simulink model "aero_guidance_airframe"  (Simulink 6.0)
settings: Solver=ode45  SolverMode=SingleTasking  StartTime=0.0  StopTime=10.0  RelTol=1e-3  AbsTol=1e-6
PreLoadFcn:
  | aero_guid_dat
values from neighbouring files (symbols this model uses):
  alpha_vec = [-20:1:20]'*d2r    [aero_guid_dat.m]
  Cm_el = -0.206000/d2r    (= -11.8029305797)    [aero_guid_dat.m]
  Cm_q = -1.719    [aero_guid_dat.m]
  Cz_el = -0.034000/d2r    (= -1.94805650344)    [aero_guid_dat.m]
  d_ref = 0.75/m2ft    (= 0.228599992685)    [aero_guid_dat.m]
  g = 9.81    [aero_guid_dat.m]    (also in aero_raddat.m = 32.2; f14dat.m = 32.2; f14dat_digital.m = 32.2)
  h_ini = 10000/m2ft    (= 3047.99990246)    [aero_guid_dat.m]    (also in aero_lin_aero.m = 10000/m2ft)
  Mach_vec = [2:0.5:4]    [aero_guid_dat.m]
  S_ref = 0.44/m2ft^2    (= 0.0408773349839)    [aero_guid_dat.m]
  Thrust = 10e3    (= 10000)    [aero_guid_dat.m]
  x_ini = 0    [aero_guid_dat.m]
libraries: aerospace x3, simulink x3
settings Model: Creator=The MathWorks Inc.  LastModifiedBy=batserve  ExtModeTrigMode=oneshot  ExtModeArmWhenConnect=off  ExtModeAutoUpdateStatusClock=off
settings DataIOCC: LimitDataPoints=off  SignalLoggingName=logsOut
settings OptimizationCC: BlockReduction=off  BooleanDataType=off
settings DebuggingCC: CheckExecutionContextPreStartOutputMsg=on  CheckExecutionContextRuntimeOutputMsg=on  SolverPrmCheckMsg=none
settings HardwareCC: TargetUnknown=on
settings ModelReferenceCC: UpdateModelReferenceTargets=IfOutOfDate

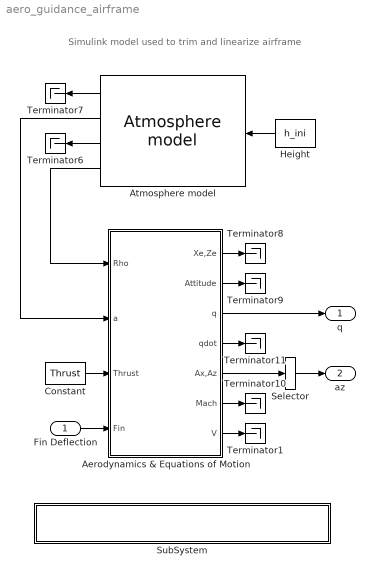
== system aero_guidance_airframe ==
  note: Simulink model used to trim and linearize airframe
  Fin Deflection : Inport  Port=1  LatchInput=off
  Aerodynamics & Equations of Motion : Subsystem  PropExecContextAcrossSSBoundary=on
  Atmosphere model : aerospace/Atmosphere/Atmosphere model  Orientation=left
  Constant : Constant  Value=Thrust
  Height : Constant  Orientation=left  Value=h_ini
  Selector : Selector  Elements=[2]  InputPortWidth=2
  SubSystem : Subsystem  PropExecContextAcrossSSBoundary=on
      settings: OpenFcn=aero_lin_aero
      mask Display: disp('Double-click here to generate linearizations')
  Terminator{1,6..11} (7 alike) : Terminator
  q : Outport  InitialOutput=0
  az : Outport  Port=2  InitialOutput=0
  wires:
  Height/1 -> Atmosphere model/1
  Atmosphere model/1 -> Terminator7/1
  Atmosphere model/3 -> Terminator6/1
  Constant/1 -> Aerodynamics & Equations of Motion/3(Thrust)
  Fin Deflection/1 -> Aerodynamics & Equations of Motion/4(Fin)
  Aerodynamics & Equations of Motion/1(Xe,Ze) -> Terminator8/1
  Aerodynamics & Equations of Motion/2(Attitude) -> Terminator9/1
  Aerodynamics & Equations of Motion/3(q) -> q/1
  Aerodynamics & Equations of Motion/4(qdot) -> Terminator11/1
  Aerodynamics & Equations of Motion/5(Ax,Az) -> Selector/1
  Aerodynamics & Equations of Motion/6(Mach) -> Terminator10/1
  Aerodynamics & Equations of Motion/7(V) -> Terminator1/1
  Atmosphere model/4 -> Aerodynamics & Equations of Motion/1(Rho)
  Atmosphere model/2 -> Aerodynamics & Equations of Motion/2(a)
  Selector/1 -> az/1

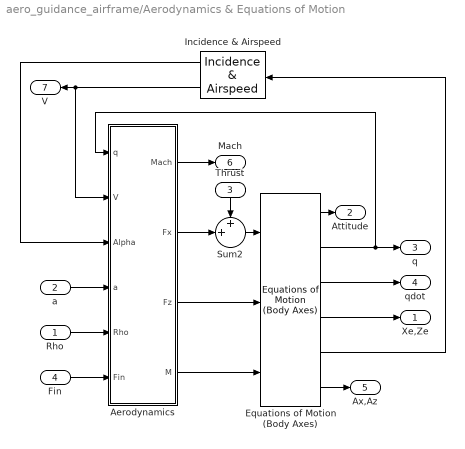
== system aero_guidance_airframe/Aerodynamics & Equations of Motion ==
  Rho : Inport  Port=1  LatchInput=off
  a : Inport  Port=2  LatchInput=off
  Thrust : Inport  Orientation=down  Port=3  LatchInput=off
  Fin : Inport  Port=4  LatchInput=off
  " Equations of Motion (Body Axes)" : aerospace/3DoF Equations of Motion / Equations of Motion (Body Axes)  v_ini=v_ini  theta_ini=theta_ini  alpha_ini=alpha_ini  q_ini=q_ini  pos_ini=[x_ini -h_ini]  mass=mass  Iyy=Iyy  g=g
  Aerodynamics : Subsystem  PropExecContextAcrossSSBoundary=on
  Incidence & Airspeed : aerospace/3DoF Equations of Motion /Incidence  & Airspeed  Orientation=left
  Sum2 : Sum  Inputs=++|  SaturateOnIntegerOverflow=on  InputSameDT=on
  Xe,Ze : Outport  InitialOutput=0
  Attitude : Outport  Port=2  InitialOutput=0
  q : Outport  Port=3  InitialOutput=0
  qdot : Outport  Port=4  InitialOutput=0
  Ax,Az : Outport  Port=5  InitialOutput=0
  Mach : Outport  Port=6  InitialOutput=0
  V : Outport  Orientation=left  Port=7  InitialOutput=0
  wires:
  " Equations of Motion (Body Axes)"/5 -> Incidence & Airspeed/1
  " Equations of Motion (Body Axes)"/6 -> Ax,Az/1
  " Equations of Motion (Body Axes)"/4 -> Xe,Ze/1
  " Equations of Motion (Body Axes)"/1 -> Attitude/1
  " Equations of Motion (Body Axes)"/3 -> qdot/1
  " Equations of Motion (Body Axes)"/2 -> Aerodynamics/1(q), q/1
  Thrust/1 -> Sum2/1
  Aerodynamics/2(Fx) -> Sum2/2
  Aerodynamics/3(Fz) -> " Equations of Motion (Body Axes)"/2
  Incidence & Airspeed/2 -> Aerodynamics/2(V), V/1
  Fin/1 -> Aerodynamics/6(Fin)
  a/1 -> Aerodynamics/4(a)
  Rho/1 -> Aerodynamics/5(Rho)
  Incidence & Airspeed/1 -> Aerodynamics/3(Alpha)
  Sum2/1 -> " Equations of Motion (Body Axes)"/1
  Aerodynamics/4(" M") -> " Equations of Motion (Body Axes)"/3
  Aerodynamics/1(" Mach") -> Mach/1

== system aero_guidance_airframe/SubSystem ==

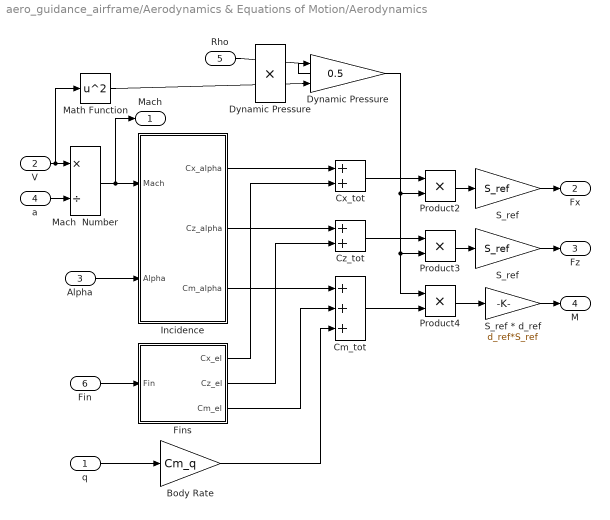
== system aero_guidance_airframe/Aerodynamics & Equations of Motion/Aerodynamics ==
  q : Inport  Port=1  LatchInput=off
  V : Inport  Port=2  LatchInput=off
  Alpha : Inport  Port=3  LatchInput=off
  a : Inport  Port=4  LatchInput=off
  Rho : Inport  Port=5  LatchInput=off
  Fin : Inport  Port=6  LatchInput=off
  Body Rate : Gain  Gain=Cm_q  SaturateOnIntegerOverflow=on
  Cm_tot : Sum  Inputs=+++  SaturateOnIntegerOverflow=on  InputSameDT=on
  Cx_tot : Sum  SaturateOnIntegerOverflow=on  InputSameDT=on
  Cz_tot : Sum  SaturateOnIntegerOverflow=on  InputSameDT=on
  Dynamic Pressure : Gain  Gain=0.5  SaturateOnIntegerOverflow=on
  Dynamic Pressure : Product  SaturateOnIntegerOverflow=on  RndMeth=Zero  InputSameDT=on
  Fins : Subsystem  PropExecContextAcrossSSBoundary=on
  Incidence : Subsystem  PropExecContextAcrossSSBoundary=on
  Mach  Number : Product  Inputs=*/  SaturateOnIntegerOverflow=on  RndMeth=Zero  InputSameDT=on
  Math Function : Math  Operator=square  SaturateOnIntegerOverflow=on
  Product2 : Product  SaturateOnIntegerOverflow=on  RndMeth=Zero  InputSameDT=on
  Product3 : Product  SaturateOnIntegerOverflow=on  RndMeth=Zero  InputSameDT=on
  Product4 : Product  SaturateOnIntegerOverflow=on  RndMeth=Zero  InputSameDT=on
  S_ref : Gain  Gain=S_ref  SaturateOnIntegerOverflow=on
  S_ref * d_ref : Gain  Gain=d_ref*S_ref  SaturateOnIntegerOverflow=on
  "S_ref " : Gain  Gain=S_ref  SaturateOnIntegerOverflow=on
  " Mach" : Outport  InitialOutput=0
  Fx : Outport  Port=2  InitialOutput=[0]
  Fz : Outport  Port=3  InitialOutput=0
  " M" : Outport  Port=4  InitialOutput=0
  wires:
  Mach  Number/1 -> " Mach"/1, Incidence/1(Mach)
  q/1 -> Body Rate/1
  Cm_tot/1 -> Product4/2
  Product4/1 -> S_ref * d_ref/1
  S_ref * d_ref/1 -> " M"/1
  Fin/1 -> Fins/1(Fin)
  "S_ref "/1 -> Fz/1
  Product3/1 -> "S_ref "/1
  S_ref/1 -> Fx/1
  Product2/1 -> S_ref/1
  Cz_tot/1 -> Product3/1
  Cx_tot/1 -> Product2/1
  Alpha/1 -> Incidence/2(Alpha)
  a/1 -> Mach  Number/2
  Body Rate/1 -> Cm_tot/3
  Fins/3(Cm_el) -> Cm_tot/2
  Incidence/3(Cm_alpha) -> Cm_tot/1
  Fins/2(Cz_el) -> Cz_tot/2
  Incidence/2(Cz_alpha) -> Cz_tot/1
  Fins/1(Cx_el) -> Cx_tot/2
  Incidence/1(Cx_alpha) -> Cx_tot/1
  V/1 -> Mach  Number/1, Math Function/1
  Dynamic Pressure/1 -> Product4/1, Product3/2, Product2/2
  Dynamic Pressure/1 -> Dynamic Pressure/1
  Rho/1 -> Dynamic Pressure/1
  Math Function/1 -> Dynamic Pressure/2

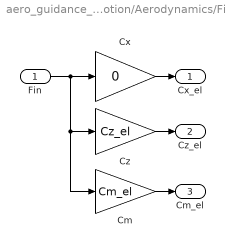
== system aero_guidance_airframe/Aerodynamics & Equations of Motion/Aerodynamics/Fins ==
  Fin : Inport  Port=1  LatchInput=off
  Cm : Gain  Gain=Cm_el  SaturateOnIntegerOverflow=on
  Cx : Gain  Gain=0  SaturateOnIntegerOverflow=on
  Cz : Gain  Gain=Cz_el  SaturateOnIntegerOverflow=on
  Cx_el : Outport  InitialOutput=0
  Cz_el : Outport  Port=2  InitialOutput=0
  Cm_el : Outport  Port=3  InitialOutput=0
  wires:
  Cz/1 -> Cz_el/1
  Cm/1 -> Cm_el/1
  Cx/1 -> Cx_el/1
  Fin/1 -> Cz/1, Cm/1, Cx/1

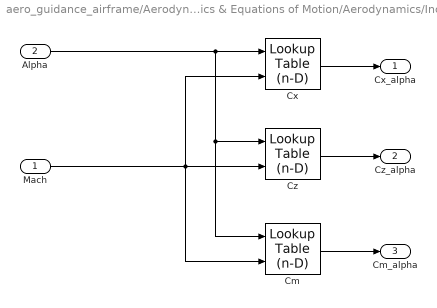
== system aero_guidance_airframe/Aerodynamics & Equations of Motion/Aerodynamics/Incidence ==
  Mach : Inport  Port=1  LatchInput=off
  Alpha : Inport  Port=2  LatchInput=off
  Cm : simulink/Lookup Tables/Lookup Table (n-D)  numDimsPopupSelect=2  bp1=alpha_vec  bp2=Mach_vec  bp3=[1:3]  bp4=[1:3]  bpcell={ [1:3], [1:3] }  explicitNumDims=2  searchMode=Binary Search  cacheBpFlag=on  vectorInputFlag=off  tableData=Cm_alpha  interpMethod=Linear  extrapMethod=Linear  rangeErrorMode=None
  Cx : simulink/Lookup Tables/Lookup Table (n-D)  numDimsPopupSelect=2  bp1=alpha_vec  bp2=Mach_vec  bp3=[1:3]  bp4=[1:3]  bpcell={ [1:3], [1:3] }  explicitNumDims=2  searchMode=Binary Search  cacheBpFlag=on  vectorInputFlag=off  tableData=Cx_alpha  interpMethod=Linear  extrapMethod=Linear  rangeErrorMode=None
  Cz : simulink/Lookup Tables/Lookup Table (n-D)  numDimsPopupSelect=2  bp1=alpha_vec  bp2=Mach_vec  bp3=[1:3]  bp4=[1:3]  bpcell={ [1:3], [1:3] }  explicitNumDims=2  searchMode=Binary Search  cacheBpFlag=on  vectorInputFlag=off  tableData=Cz_alpha  interpMethod=Linear  extrapMethod=Linear  rangeErrorMode=None
  Cx_alpha : Outport  InitialOutput=0
  Cz_alpha : Outport  Port=2  InitialOutput=0
  Cm_alpha : Outport  Port=3  InitialOutput=0
  wires:
  Cx/1 -> Cx_alpha/1
  Cz/1 -> Cz_alpha/1
  Cm/1 -> Cm_alpha/1
  Alpha/1 -> Cx/1, Cm/1, Cz/1
  Mach/1 -> Cx/2, Cm/2, Cz/2
